simulink model "ActualMessage"  (R2024a)
settings: Solver=FixedStepAuto  StartTime=0.0  StopTime=0  FixedStep=1  RelTol=1e-3  EnableMultiTasking=on
undefined symbols (not defined in the file): LED, rcd2, timestamp
libraries: RCD2 x3
settings Model: Creator=damerius  LastModifiedBy=damerius
settings SolverCC: ConcurrentTasks=on
settings DataIOCC: SaveOutput=off  SignalLogging=off  DSMLogging=off  SaveTime=off  ReturnWorkspaceOutputs=off
settings OptimizationCC: DefaultParameterBehavior=Inlined  ZeroExternalMemoryAtStartup=off  ZeroInternalMemoryAtStartup=off  SimCompilerOptimization=on
settings DebuggingCC: UnconnectedInputMsg=warning  UnconnectedOutputMsg=warning  UnconnectedLineMsg=warning
settings HardwareCC: ProdBitPerLong=64  ProdHWDeviceType=Intel->x86-64 (Linux 64)  TargetBitPerLong=64  TargetBitPerPointer=64  TargetBitPerSizeT=64  TargetBitPerPtrDiffT=64  TargetLargestAtomicFloat=Float  TargetIntDivRoundTo=Zero  TargetEndianess=LittleEndian  TargetWordSize=64  TargetHWDeviceType=Intel->x86-64 (Linux 64)  ProdEqTarget=off
settings ModelReferenceCC: EnableRefExpFcnMdlSchedulingChecks=on
settings SFSimCC: SimParseCustomCode=off  SimGenImportedTypeDefs=on  SimTargetLang=C++
settings RTWCC: GenCodeOnly=on  PackageGeneratedCodeAndArtifacts=on  PackageName=PackNGo  BuildConfiguration=Faster Runs  TargetLang=C++
settings CodeAppCC: ForceParamTrailComments=on  MaxIdLength=128  StateflowObjectComments=on  MATLABSourceComments=on  UseSimReservedNames=on
settings GRTTargetCC: TargetLangStandard=C++11 (ISO)  MatFileLogging=off  CodeInterfacePackaging=C++ class

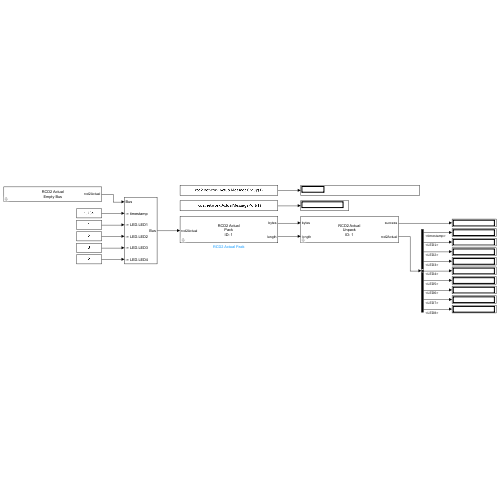
[thumbnail: Simulink's stored preview of the top-level diagram]
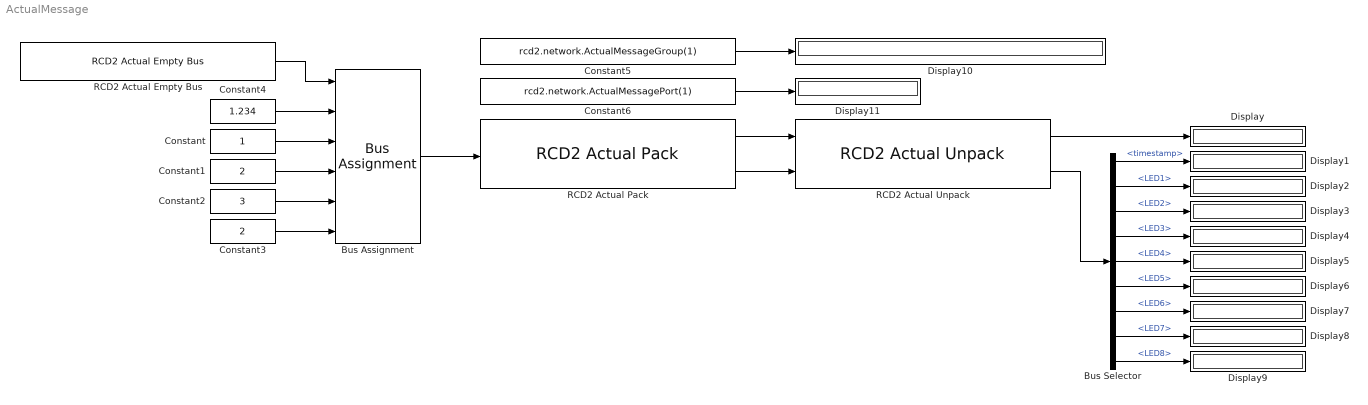
== system ActualMessage ==
  Bus Assignment : BusAssignment  AssignedSignals=timestamp,LED.LED1,LED.LED2,LED.LED3,LED.LED4
  Bus Selector : BusSelector  OutputSignals=timestamp,LED.LED1,LED.LED2,LED.LED3,LED.LED4,LED.LED5,LED.LED6,LED.LED7,LED.LED8
  Constant : Constant  OutDataTypeStr=uint8
  Constant1 : Constant  Value=2  OutDataTypeStr=uint8
  Constant2 : Constant  Value=3  OutDataTypeStr=uint8
  Constant3 : Constant  Value=2  OutDataTypeStr=uint8
  Constant4 : Constant  Value=1.234  OutDataTypeStr=double
  Constant5 : Constant  Value=rcd2.network.ActualMessageGroup(1)
  Constant6 : Constant  Value=rcd2.network.ActualMessagePort(1)
  Display{,1..11} (12 alike) : Display
  RCD2 Actual Empty Bus : RCD2/From RCD2/RCD2 Actual Empty Bus
      settings: SourceProductName=Remote Control Device 2
  RCD2 Actual Pack : RCD2/From RCD2/RCD2 Actual Pack  idRCD=1
      settings: SourceProductName=Remote Control Device 2
  RCD2 Actual Unpack : RCD2/From RCD2/RCD2 Actual Unpack  idRCD=1
      settings: SourceProductName=Remote Control Device 2
  wires:
  RCD2 Actual Pack/1 -> RCD2 Actual Unpack/1
  RCD2 Actual Pack/2 -> RCD2 Actual Unpack/2
  RCD2 Actual Unpack/1 -> Display/1
  RCD2 Actual Empty Bus/1 -> Bus Assignment/1
  Constant4/1 -> Bus Assignment/2
  Constant/1 -> Bus Assignment/3
  Constant1/1 -> Bus Assignment/4
  Constant2/1 -> Bus Assignment/5
  Constant3/1 -> Bus Assignment/6
  Bus Assignment/1 -> RCD2 Actual Pack/1
  RCD2 Actual Unpack/2 -> Bus Selector/1
  Bus Selector/1 -> Display1/1  "<timestamp>"
  Bus Selector/2 -> Display2/1  "<LED1>"
  Bus Selector/3 -> Display3/1  "<LED2>"
  Bus Selector/5 -> Display5/1  "<LED4>"
  Bus Selector/4 -> Display4/1  "<LED3>"
  Bus Selector/8 -> Display8/1  "<LED7>"
  Bus Selector/9 -> Display9/1  "<LED8>"
  Bus Selector/7 -> Display7/1  "<LED6>"
  Bus Selector/6 -> Display6/1  "<LED5>"
  Constant5/1 -> Display10/1
  Constant6/1 -> Display11/1
